simulink model "CruiseControl_IntCalcFix"  (R2015a)
settings: Solver=FixedStepDiscrete  StartTime=0.0  StopTime=16  FixedStep=0.1  RelTol=1e-3
PreLoadFcn:
  | CruiseControl_DivByZero_dd;
model workspace (MAT data in the model file):
  min_throttle = 0.6
  min_speed = 20
values from neighbouring files (symbols this model uses):
  holdrate = mpt.Parameter    [CruiseControl_DivByZero_dd.m]
  incdec = mpt.Parameter    [CruiseControl_DivByZero_dd.m]
  maxtspeed = mpt.Parameter    [CruiseControl_DivByZero_dd.m]
  mintspeed = mpt.Parameter    [CruiseControl_DivByZero_dd.m]
settings Model: RecordCoverage=on  CovMetricSettings=dcme  CovHtmlReporting=off  covSaveCumulativeToWorkspaceVar=off  CovSaveSingleToWorkspaceVar=off  CovSFcnEnable=off  Creator=The MathWorks Inc.  LastModifiedBy=colosky
settings DataIOCC: SaveOutput=off  SaveTime=off
settings OptimizationCC: InlineParams=on  InlineInvariantSignals=on  ExpressionDepthLimit=2147483647  InitFltsAndDblsToZero=on
settings DebuggingCC: SaveWithParameterizedLinksMsg=none  UnderspecifiedInitializationDetection=Classic  MergeDetectMultiDrivingBlocksExec=none  SolverPrmCheckMsg=warning  FcnCallInpInsideContextMsg=UseLocalSettings  StateNameClashWarn=warning  StrictBusMsg=ErrorOnBusTreatedAsVector
settings SFSimCC: SimParseCustomCode=off
settings GRTTargetCC: TargetFcnLib=ansi_tfl_tmw.mat  CombineOutputUpdateFcns=off  GRTInterface=on
settings ConfigComp: Description=Design Verifier Custom Configuration Component  DVMode=DesignErrorDetection  DVMaxProcessTime=3000  DVDisplayUnsatisfiableObjectives=on  DVAutomaticStubbing=off  DVMakeOutputFilesUnique=off  DVParametersConfigFileName=C:\matlab_user\Temp\MAC_MASTER\VnV_MASTER_MAC\Models\DesignErrDetect\CruiseControl_SLDV_ParTable.m  DVModelCoverageObjectives=MCDC  DVMaxTestCaseSteps=500  DVTestSuiteOptimization=CombinedObjectives  DVAssertions=EnableAll  DVProofAssumptions=EnableAll  DVDetectIntegerOverflow=off  DVDetectDeadLogic=on  DVDetectActiveLogic=on  DVMaxViolationSteps=50  DVSaveDataFile=off  DVSaveHarnessModel=on  DVModelReferenceHarness=on  DVReportIncludeGraphics=on

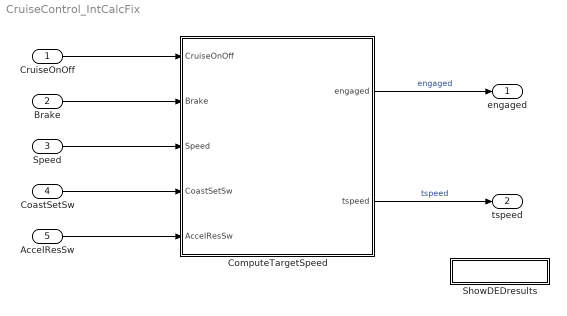
== system CruiseControl_IntCalcFix ==
  CruiseOnOff : Inport  OutDataTypeStr=boolean  PortDimensions=1
  Brake : Inport  Port=2  OutDataTypeStr=boolean  PortDimensions=1
  Speed : Inport  Port=3  OutDataTypeStr=single  PortDimensions=1
  CoastSetSw : Inport  Port=4  OutDataTypeStr=boolean  PortDimensions=1
  AccelResSw : Inport  Port=5  OutDataTypeStr=boolean  PortDimensions=1
  ComputeTargetSpeed : Stateflow chart  TreatAsAtomicUnit=on
  ShowDEDresults : Subsystem
      settings: OpenFcn=|
      | p = slproject.getCurrentProject;
      | sldvhighlight(bdroot, ...
      | fullfile(p.RootFolder,'Models\DesignErrDetect', ...
      |     [bdroot '_sldvdata_Results.mat']));
      | clear p
      mask Display: disp(['Show DED Results']);
  engaged : Outport
  tspeed : Outport  Port=2
  wires:
  ComputeTargetSpeed/2(tspeed) -> tspeed/1  "tspeed"
  ComputeTargetSpeed/1(engaged) -> engaged/1  "engaged"
  AccelResSw/1 -> ComputeTargetSpeed/5(AccelResSw)
  CruiseOnOff/1 -> ComputeTargetSpeed/1(CruiseOnOff)
  Brake/1 -> ComputeTargetSpeed/2(Brake)
  CoastSetSw/1 -> ComputeTargetSpeed/4(CoastSetSw)
  Speed/1 -> ComputeTargetSpeed/3(Speed)

== system CruiseControl_IntCalcFix/ShowDEDresults ==

== stateflow chart CruiseControl_IntCalcFix/ComputeTargetSpeed ==
  state OFF
    en:
    engaged = false;
    tspeed = 0;
  state CRUISE
    state ON
      en: engaged = true;
      state Accel
        tspeed = tspeed + incdec;
      state Steady
      state Coast
        tspeed = tspeed - incdec;
      (junction 60) -> Accel
      (junction 57) -> (junction 60) : [after(incdec*uint8(10)...
          | /holdrate,tick)]
      Accel -> (junction 57) [order 2]
      Steady -> Accel [order 1] : [hasChangedTo(AccelResSw,true) ...
          | && tspeed < maxtspeed]
      Accel -> Steady [order 1] : [!AccelResSw || ...
          | tspeed > maxtspeed]
      Steady -> (junction 75) [order 3] : [hasChangedTo(CoastSetSw,true)]
      (default) -> (junction 75)
      (junction 75) -> (junction 77) : {tspeed = Speed;}
      (junction 77) -> Steady
      Steady -> Coast [order 2] : [hasChangedTo(CoastSetSw,true) ...
          | && tspeed > mintspeed]
      Coast -> Steady [order 1] : [!CoastSetSw || ...
          | tspeed < mintspeed]
      (junction 72) -> Coast
      (junction 71) -> (junction 72) : [after(incdec*uint8(10)...
          | /holdrate,tick)]
      Coast -> (junction 71) [order 2]
    state STANDBY
      en:
      engaged=false;
    (default) -> STANDBY
    ON -> STANDBY : [Brake||Speed> maxtspeed||Speed<mintspeed]
    STANDBY -> (junction 103) : [~Brake && ...
        | Speed<=maxtspeed && ...
        | Speed>=mintspeed]
    (junction 103) -> Steady [order 1] : [hasChangedTo(AccelResSw,true)...
        | &&tspeed!=0]
    (junction 103) -> (junction 106) [order 2]
    (junction 106) -> ON : [hasChangedTo(CoastSetSw,true)]
  (default) -> OFF
  OFF -> CRUISE : [CruiseOnOff]
  CRUISE -> OFF : [~CruiseOnOff]
  data: engaged output boolean; CruiseOnOff input; Brake input; Speed input; CoastSetSw input; AccelResSw input; tspeed output single; incdec parameter; holdrate parameter; maxtspeed parameter; mintspeed parameter
